simulink model "diskr"  (Simulink 7.6)
settings: Solver=ode45  StartTime=0.0  StopTime=1800.0  RelTol=1e-3
values from neighbouring files (symbols this model uses):
  A = 0.00278    [koef.m]
  A12 = 18.54e-6    (= 1.854e-05)    [koef.m]
  A23 = 17.5e-6    (= 1.75e-05)    [koef.m]
  A34 = 18.75e-6    (= 1.875e-05)    [koef.m]
  A4 = 13.44e-6    (= 1.344e-05)    [koef.m]
  g = 9.81    [koef.m]
  H = c2d(G_par,T_a,'tustin')    [koef.m]
  hmax = 0.338    [koef.m]
  T_n = 127    [koef.m]
  T_v = 12.7    [koef.m]
settings Model: Creator=Johannes  LastModifiedBy=Johannes

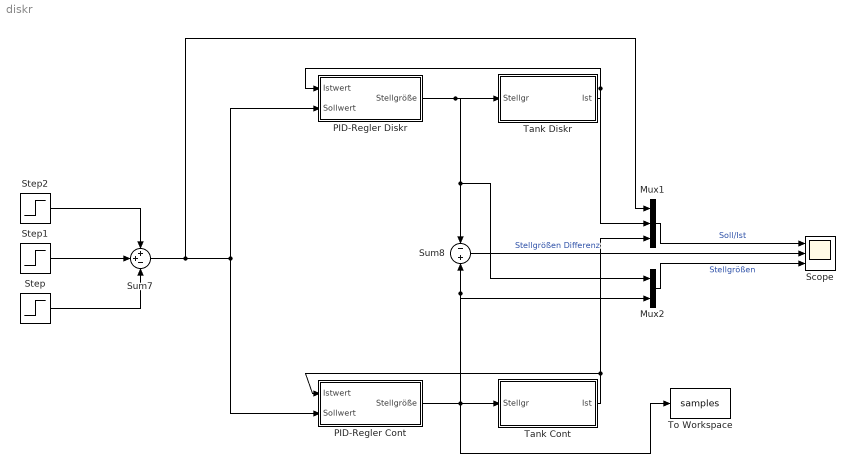
== system diskr ==
  Mux1 : Mux  Inputs=3
  Mux2 : Mux  Inputs=2
  PID-Regler Cont : Subsystem
  PID-Regler Diskr : Subsystem
  Scope : Scope  NumInputPorts=3
      settings: YMin=0~0.04~1.35e+010  YMax=1.9e+010~0.115~1.825e+010  SampleInput=on  SampleTime=1
  Step : Step  Time=600  After=0.5*0.0338  SampleTime=0
  Step1 : Step  After=2.5*0.0338  SampleTime=0
  Step2 : Step  Time=1200  After=1*0.0338  SampleTime=0
  Sum7 : Sum  Inputs=++-
  Sum8 : Sum  Inputs=-|+
  Tank Cont : Subsystem
  Tank Diskr : Subsystem
  To Workspace : ToWorkspace  VariableName=samples  SampleTime=60  SaveFormat=Array
  wires:
  Step/1 -> Sum7/3
  Mux1/1 -> Scope/1  "Soll/Ist"
  Step1/1 -> Sum7/2
  Step2/1 -> Sum7/1
  PID-Regler Diskr/1(Stellgröße) -> Tank Diskr/1(Stellgr), Sum8/1, Mux2/1
  PID-Regler Cont/1(Stellgröße) -> Tank Cont/1(Stellgr), Mux2/2, Sum8/2, To Workspace/1
  Tank Diskr/1(Ist) -> PID-Regler Diskr/1(Istwert), Mux1/2
  Tank Cont/1(Ist) -> PID-Regler Cont/1(Istwert), Mux1/3
  Sum7/1 -> PID-Regler Cont/2(Sollwert), PID-Regler Diskr/2(Sollwert), Mux1/1
  Sum8/1 -> Scope/2  "Stellgrößen Differenz"
  Mux2/1 -> Scope/3  "Stellgrößen"

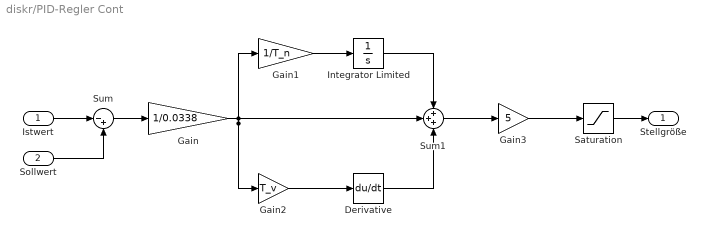
== system diskr/PID-Regler Cont ==
  Istwert : Inport
  Sollwert : Inport  Port=2
  Derivative : Derivative
  Gain : Gain  Gain=1/0.0338
  Gain1 : Gain  Gain=1/T_n
  Gain2 : Gain  Gain=T_v
  Gain3 : Gain  Gain=5
  Integrator Limited : Integrator  LimitOutput=on  UpperSaturationLimit=10  LowerSaturationLimit=0
  Saturation : Saturate  UpperLimit=10  LowerLimit=0
  Sum : Sum  Inputs=|-+
  Sum1 : Sum  Inputs=+++
  Stellgröße : Outport
  wires:
  Istwert/1 -> Sum/1
  Sollwert/1 -> Sum/2
  Sum/1 -> Gain/1
  Gain/1 -> Gain1/1, Gain2/1, Sum1/2
  Gain2/1 -> Derivative/1
  Gain1/1 -> Integrator Limited/1
  Integrator Limited/1 -> Sum1/1
  Derivative/1 -> Sum1/3
  Sum1/1 -> Gain3/1
  Gain3/1 -> Saturation/1
  Saturation/1 -> Stellgröße/1

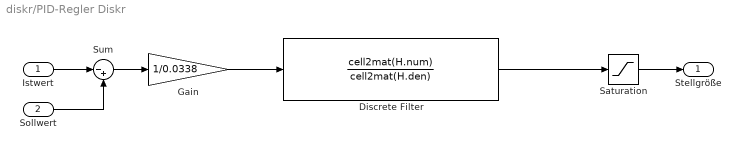
== system diskr/PID-Regler Diskr ==
  Istwert : Inport
  Sollwert : Inport  Port=2
  Discrete Filter : DiscreteFilter  Numerator=cell2mat(H.num)  Denominator=cell2mat(H.den)  SampleTime=H.Ts
  Gain : Gain  Gain=1/0.0338
  Saturation : Saturate  UpperLimit=10  LowerLimit=0
  Sum : Sum  Inputs=|-+
  Stellgröße : Outport
  wires:
  Istwert/1 -> Sum/1
  Sollwert/1 -> Sum/2
  Sum/1 -> Gain/1
  Gain/1 -> Discrete Filter/1
  Saturation/1 -> Stellgröße/1
  Discrete Filter/1 -> Saturation/1

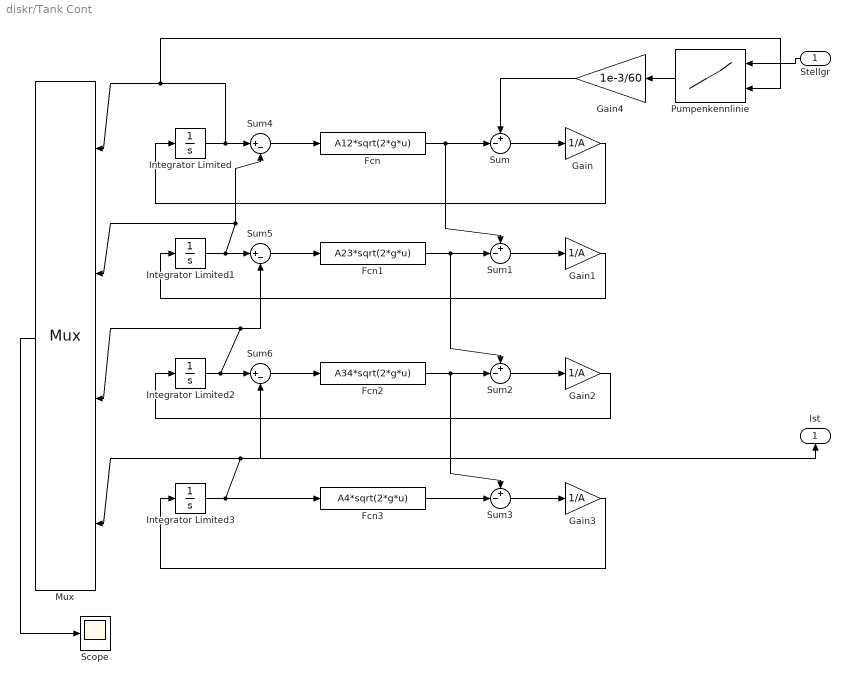
== system diskr/Tank Cont ==
  Stellgr : Inport
  Fcn : Fcn  Expr=A12*sqrt(2*g*u)
  Fcn1 : Fcn  Expr=A23*sqrt(2*g*u)
  Fcn2 : Fcn  Expr=A34*sqrt(2*g*u)
  Fcn3 : Fcn  Expr=A4*sqrt(2*g*u)
  Gain{,1..3} (4 alike) : Gain  Gain=1/A
  Gain4 : Gain  Gain=1e-3/60
  Integrator Limited{,1..3} (4 alike) : Integrator  LimitOutput=on  UpperSaturationLimit=hmax  LowerSaturationLimit=0
  Mux : Mux
      settings: DisplayOption=signals
  Pumpenkennlinie : Lookup2D  RowIndex=[ 0 2 3.5 4 6 8 10 12]  ColumnIndex=[ 0 1 2 3 4 5 6 7 8 9 10]*0.338/10  Table=[ 0 0 0 0 0 0 0 0 0 0 0 ; 0 0 0 0 0 0 0 0 0 0 0 ; 0.3373 0.2611 0.1115 0.0311 0 0 0 0 0 0 0 ; 0.6051 0.5588 0.5222 0.4851 0.4488 0.3499 0.2844 0.2148 0.1899 0.1431 0.0861; 1.3367 1.3073 1.2845 1.2640 1.2531 1.2297 1.2081 1.1914 1.1831 1.1704 1.1614 ; 1.8718 1.8689 1.8632 1.8579 1.8491 1.8375 1.8271 1.8120 1.8045 1.7843 1.7733 ; 2.4327 2.4253 2.4193 2.4161 2.4095 2.4071 2.4035 2.3993 2.3941 2.3847 2.3799 ; 2.9356 2.9306 2.9291 2.9187 2.9165 2.9125 2.8945 2.8922 2.8855 2.8775 2.8744 ]  SaturateOnIntegerOverflow=on  InputSameDT=on
  Scope : Scope
      settings: SaveName=ScopeData2
  Sum{,1..3} (4 alike) : Sum  Inputs=+-|
  Sum4 : Sum  Inputs=|+-
  Sum5 : Sum  Inputs=|+-
  Sum6 : Sum  Inputs=|+-
  Ist : Outport
  wires:
  Fcn/1 -> Sum/2, Sum1/1
  Fcn1/1 -> Sum1/2, Sum2/1
  Fcn2/1 -> Sum2/2, Sum3/1
  Fcn3/1 -> Sum3/2
  Sum/1 -> Gain/1
  Sum1/1 -> Gain1/1
  Sum2/1 -> Gain2/1
  Sum3/1 -> Gain3/1
  Gain/1 -> Integrator Limited/1
  Integrator Limited/1 -> Sum4/1, Mux/1, Pumpenkennlinie/2
  Sum4/1 -> Fcn/1
  Integrator Limited1/1 -> Sum5/1, Sum4/2, Mux/2
  Sum5/1 -> Fcn1/1
  Integrator Limited2/1 -> Sum6/1, Sum5/2, Mux/3
  Sum6/1 -> Fcn2/1
  Integrator Limited3/1 -> Sum6/2, Mux/4, Ist/1, Fcn3/1
  Gain1/1 -> Integrator Limited1/1
  Gain2/1 -> Integrator Limited2/1
  Gain3/1 -> Integrator Limited3/1
  Gain4/1 -> Sum/1
  Mux/1 -> Scope/1
  Pumpenkennlinie/1 -> Gain4/1
  Stellgr/1 -> Pumpenkennlinie/1

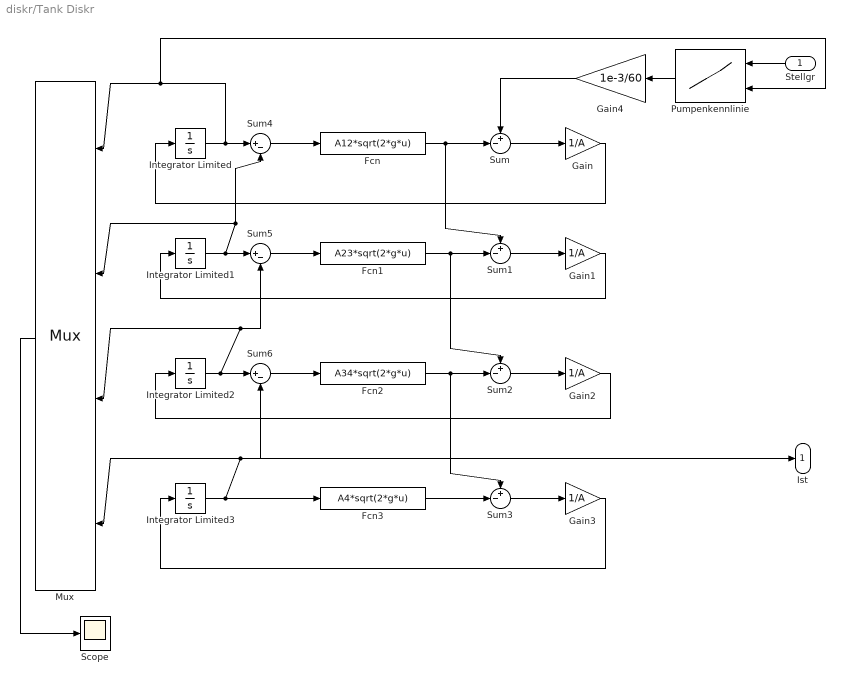
== system diskr/Tank Diskr ==
  Stellgr : Inport
  Fcn : Fcn  Expr=A12*sqrt(2*g*u)
  Fcn1 : Fcn  Expr=A23*sqrt(2*g*u)
  Fcn2 : Fcn  Expr=A34*sqrt(2*g*u)
  Fcn3 : Fcn  Expr=A4*sqrt(2*g*u)
  Gain{,1..3} (4 alike) : Gain  Gain=1/A
  Gain4 : Gain  Gain=1e-3/60
  Integrator Limited{,1..3} (4 alike) : Integrator  LimitOutput=on  UpperSaturationLimit=hmax  LowerSaturationLimit=0
  Mux : Mux
      settings: DisplayOption=signals
  Pumpenkennlinie : Lookup2D  RowIndex=[ 0 2 3.5 4 6 8 10 12]  ColumnIndex=[ 0 1 2 3 4 5 6 7 8 9 10]*0.338/10  Table=[ 0 0 0 0 0 0 0 0 0 0 0 ; 0 0 0 0 0 0 0 0 0 0 0 ; 0.3373 0.2611 0.1115 0.0311 0 0 0 0 0 0 0 ; 0.6051 0.5588 0.5222 0.4851 0.4488 0.3499 0.2844 0.2148 0.1899 0.1431 0.0861; 1.3367 1.3073 1.2845 1.2640 1.2531 1.2297 1.2081 1.1914 1.1831 1.1704 1.1614 ; 1.8718 1.8689 1.8632 1.8579 1.8491 1.8375 1.8271 1.8120 1.8045 1.7843 1.7733 ; 2.4327 2.4253 2.4193 2.4161 2.4095 2.4071 2.4035 2.3993 2.3941 2.3847 2.3799 ; 2.9356 2.9306 2.9291 2.9187 2.9165 2.9125 2.8945 2.8922 2.8855 2.8775 2.8744 ]  SaturateOnIntegerOverflow=on  InputSameDT=on
  Scope : Scope
      settings: SaveName=ScopeData2
  Sum{,1..3} (4 alike) : Sum  Inputs=+-|
  Sum4 : Sum  Inputs=|+-
  Sum5 : Sum  Inputs=|+-
  Sum6 : Sum  Inputs=|+-
  Ist : Outport
  wires:
  Stellgr/1 -> Pumpenkennlinie/1
  Pumpenkennlinie/1 -> Gain4/1
  Mux/1 -> Scope/1
  Gain4/1 -> Sum/1
  Gain3/1 -> Integrator Limited3/1
  Gain2/1 -> Integrator Limited2/1
  Gain1/1 -> Integrator Limited1/1
  Integrator Limited3/1 -> Fcn3/1, Ist/1, Mux/4, Sum6/2
  Sum6/1 -> Fcn2/1
  Integrator Limited2/1 -> Mux/3, Sum5/2, Sum6/1
  Sum5/1 -> Fcn1/1
  Integrator Limited1/1 -> Mux/2, Sum4/2, Sum5/1
  Sum4/1 -> Fcn/1
  Integrator Limited/1 -> Pumpenkennlinie/2, Mux/1, Sum4/1
  Gain/1 -> Integrator Limited/1
  Sum3/1 -> Gain3/1
  Sum2/1 -> Gain2/1
  Sum1/1 -> Gain1/1
  Sum/1 -> Gain/1
  Fcn3/1 -> Sum3/2
  Fcn2/1 -> Sum3/1, Sum2/2
  Fcn1/1 -> Sum2/1, Sum1/2
  Fcn/1 -> Sum1/1, Sum/2
